simulink model "testDLH_Khanhpro"  (R2022a)
settings: Solver=FixedStepAuto  StartTime=0.0  StopTime=10.0  FixedStep=0.01  RelTol=1e-3
libraries: simulink_extras x4
settings Model: Creator=Vũ Quốc Khánh  LastModifiedBy=Vũ Quốc Khánh

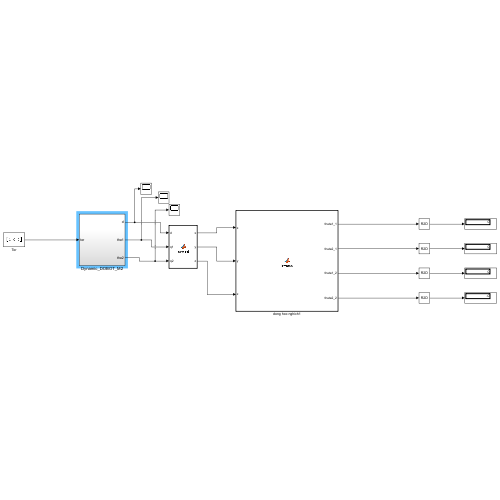
[thumbnail: Simulink's stored preview of the top-level diagram]
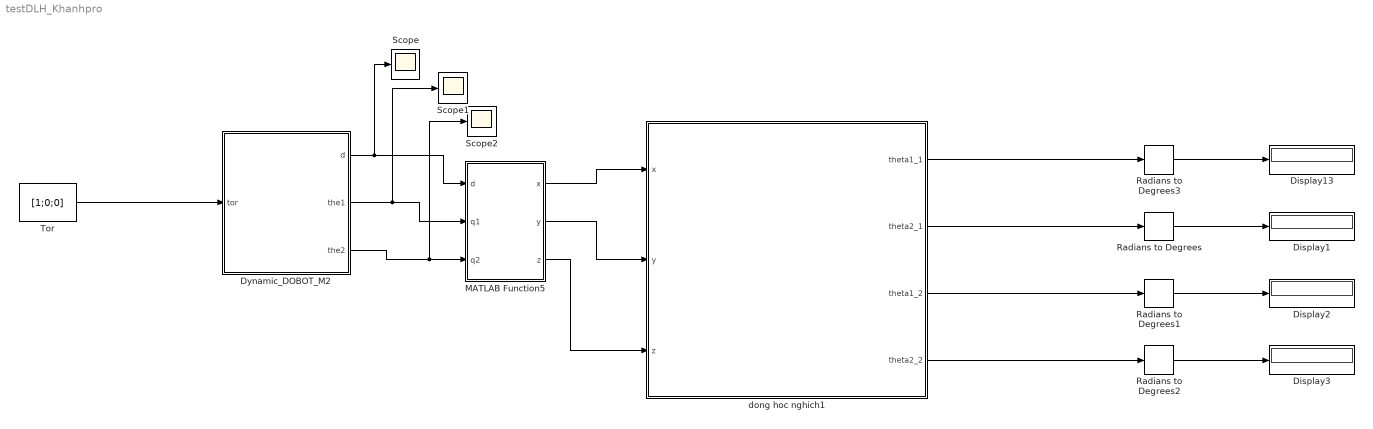
== system testDLH_Khanhpro ==
  Display{1..3,13} (4 alike) : Display
  Dynamic_DOBOT_M2 : Subsystem
  MATLAB Function5 : MATLAB Function  TreatAsAtomicUnit=on
  Radians to Degrees{,1..3} (4 alike) : simulink_extras/Transformations/Radians to Degrees
  Scope : Scope
  Scope1 : Scope
  Scope2 : Scope
  Tor : Constant  Value=[1;0;0]
  dong hoc nghich1 : MATLAB Function  TreatAsAtomicUnit=on
  wires:
  Tor/1 -> Dynamic_DOBOT_M2/1(tor)
  Dynamic_DOBOT_M2/2(the1) -> Scope1/1, MATLAB Function5/2(q1)
  Dynamic_DOBOT_M2/1(d) -> Scope/1, MATLAB Function5/1(d)
  MATLAB Function5/1(x) -> dong hoc nghich1/1(x)
  MATLAB Function5/2(y) -> dong hoc nghich1/2(y)
  MATLAB Function5/3(z) -> dong hoc nghich1/3(z)
  dong hoc nghich1/2(theta2_1) -> Radians to Degrees/1
  dong hoc nghich1/3(theta1_2) -> Radians to Degrees1/1
  dong hoc nghich1/1(theta1_1) -> Radians to Degrees3/1
  dong hoc nghich1/4(theta2_2) -> Radians to Degrees2/1
  Radians to Degrees1/1 -> Display2/1
  Radians to Degrees/1 -> Display1/1
  Radians to Degrees2/1 -> Display3/1
  Radians to Degrees3/1 -> Display13/1
  Dynamic_DOBOT_M2/3(the2) -> Scope2/1, MATLAB Function5/3(q2)

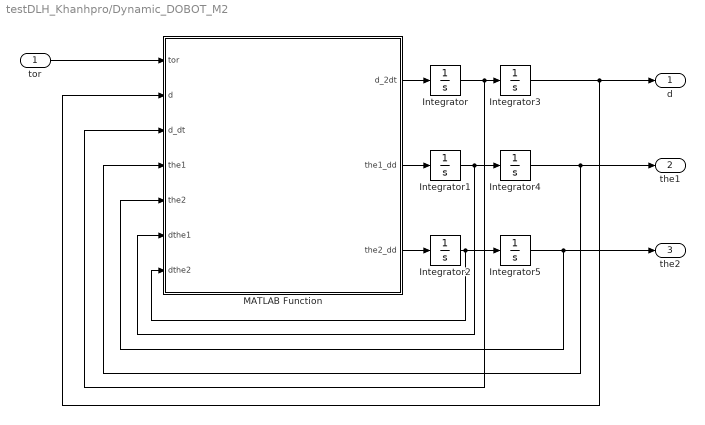
== system testDLH_Khanhpro/Dynamic_DOBOT_M2 ==
  tor : Inport
  Integrator{,1..5} (6 alike) : Integrator
  MATLAB Function : MATLAB Function  TreatAsAtomicUnit=on
  d : Outport  VectorParamsAs1DForOutWhenUnconnected=off
  the1 : Outport  Port=2  VectorParamsAs1DForOutWhenUnconnected=off
  the2 : Outport  Port=3  VectorParamsAs1DForOutWhenUnconnected=off
  wires:
  MATLAB Function/2(the1_dd) -> Integrator1/1
  Integrator4/1 -> MATLAB Function/4(the1), the1/1
  MATLAB Function/3(the2_dd) -> Integrator2/1
  Integrator/1 -> Integrator3/1, MATLAB Function/3(d_dt)
  Integrator3/1 -> MATLAB Function/2(d), d/1
  Integrator1/1 -> Integrator4/1, MATLAB Function/6(dthe1)
  Integrator2/1 -> Integrator5/1, MATLAB Function/7(dthe2)
  MATLAB Function/1(d_2dt) -> Integrator/1
  Integrator5/1 -> MATLAB Function/5(the2), the2/1
  tor/1 -> MATLAB Function/1(tor)

== matlab function testDLH_Khanhpro/Dynamic_DOBOT_M2/MATLAB Function ==
  data: tor input; d_2dt output; d input; d_dt input; the1 input; the2 input; dthe1 input; dthe2 input; the1_dd output; the2_dd output
function [d_2dt, the1_dd, the2_dd] = Dynamic(tor,d, d_dt,the1, the2, dthe1, dthe2)
m1=1; m2=1; m3=1;
L1=1; L2=1; L3=1;
g=9.81;
% MA Tran M
M11=m1+m2+m3;
M12=0;
M13=0;
M21=0;
M22=L2*L2*m2+L2*L2*m3+L3*L3*m3+2*L2*L3*m3*cos(the2);
M23=L3*m3*(L3+L2*cos(the2));
M31=0;
M32=L3*m3*(L3+L2*cos(the2));
M33=L3*L3*m3;
% Ma tran V
V11=0; 
V12= -L2*L3*dthe2*m3*sin(the2)*(2*dthe1+dthe2);
V13= L2*L3*the1*the1*m3*sin(the2);

% Ma tran G
G11=g*(m1+m2+m3);
G12=0;
G13=0;

M= [ M11,   M12,    M13;
     M21,   M22,    M23;
     M31,   M32,    M33;];
V=[V11; 
   V12;
   V13;];
G=[G11;
    G12;
    G13;];
the_dd=pinv(M)*(tor-G-V);
d_2dt=the_dd(1);
the1_dd=the_dd(2);
the2_dd=the_dd(3);
end

== matlab function testDLH_Khanhpro/dong hoc nghich1 ==
  data: x input; theta1_1 output; y input; z input; theta2_1 output; theta1_2 output; theta2_2 output
%%function [theta1, theta2] = Inverse(x,y,z)
    %%L1=1; 
   %% L2=1; 
    %%L3=1;
        %% theta2:
    %%c2=((x-L1)^2+y^2-L3^2-L1^2)/(2*L2*L3);
    % Bo nghiem 1
    %%for i=1:2
   %%     if i==1
     %%     s2=sqrt(1-c2^2);
    %%    else
   %%       s2=-sqrt(1-c2^2);
   %% end
    %%theta2=atan2(s2,c2);
   %% c1=((x-L1)*(L3*cos(theta2)+L2)+y*L3*sin(theta2))/((L3*cos(theta2)+L2)*(L3*cos(theta2)+L2)+(L3*sin(theta2))^2);
    %%s1=((L3*cos(theta2)+L2)*y -(x-L1)*L3*sin(theta2))/((L3*cos(theta2)+L2)*(L3*cos(theta2)+L2)+(L3*sin(theta2))^2);
    %%fprintf('Bo nghiem: %d ',i);
    %%theta2
    %%theta1=atan2(s1,c1)
    %%d=z

function [theta1_1, theta2_1, theta1_2, theta2_2] = Inverse(x, y, z)
    
    % Định nghĩa các hằng số
    L1 = 1; 
    L2 = 1; 
    L3 = 1;

    % Tính c2 cho theta2
    c2 = ((x - L1)^2 + y^2 - L3^2 - L2^2) / (2 * L2 * L3);
    

    % Khởi tạo các biến đầu ra cho các nghiệm
    theta1 = zeros(1, 2);
    theta2 = zeros(1, 2);
    
    for i = 1:2
        % Chọn giá trị phù hợp cho s2
        if i == 1
            s2 = sqrt(1 - c2^2);
        else
            s2 = -sqrt(1 - c2^2);
        end
        
        % Tính theta2 dựa vào s2 và c2
        theta2(i) = atan2(s2, c2);
        
        % Tính theta1 dựa vào theta2
        c1 = ((x - L1) * (L3 * cos(theta2(i)) + L2) + y * L3 * sin(theta2(i))) / ...
             ((L3 * cos(theta2(i)) + L2)^2 + (L3 * sin(theta2(i)))^2);
        s1 = ((L3 * cos(theta2(i)) + L2) * y - (x - L1) * L3 * sin(theta2(i))) / ...
             ((L3 * cos(theta2(i)) + L2)^2 + (L3 * sin(theta2(i)))^2);
        
        % Tính theta1
        theta1(i) = atan2(s1, c1);
        
        % Hiển thị kết quả
        %fprintf('Nghiệm %d: theta1 = %.4f, theta2 = %.4f\n', i, theta1(i), theta2(i));
    end
    
    % Gán các giá trị đầu ra tương ứng với hai bộ nghiệm
    theta1_1 = theta1(1);
    theta2_1 = theta2(1);
    theta1_2 = theta1(2);
    theta2_2 = theta2(2);
end

== matlab function testDLH_Khanhpro/MATLAB Function5 ==
  data: d input; q1 input; x output; q2 input; y output; z output
function [x,y,z] = forward(d,q1,q2)
%% Khai bao bien
l1=1;
l2=1;
l3=1;
x=l1 + l2*cosd(q1) + l3* ((cosd(q1)*cosd(q2))-sind(q1)*sind(q2));
y= cosd(q1)*l3*sind(q2) + sind(q1)*(l2+l3*cosd(q2));
z=d;
%%diem dau cuoi
